simulink model "v2021_10_27_modello_calcolo_trim_1_semplificato"  (R2020b)
settings: Solver=ode4  StartTime=0.0  StopTime=0.01  FixedStep=0.01  RelTol=1e-3
values from neighbouring files (symbols this model uses):
  alphavec_rad = deg2rad(alphavec)    [v2021_10_27_calcoloAerodinamica.m]
  b = 2.62    [v2021_10_27_calcoloAerodinamica.m]
  betavec_rad = deg2rad(betavec)    [v2021_10_27_calcoloAerodinamica.m]
  c = .32    (= 0.32)    [v2021_10_27_calcoloAerodinamica.m]
  cbar = .32    (= 0.32)    [v2021_10_27_calcoloAerodinamica.m]
  CD0 = 0.024    [v2021_10_27_calcoloAerodinamica.m]
  Clp = -0.5058    [v2021_10_27_calcoloAerodinamica.m]
  CLq = 19.166    [v2021_10_27_calcoloAerodinamica.m]
  Clr = 0.1459    [v2021_10_27_calcoloAerodinamica.m]
  Cmq = -81.796    [v2021_10_27_calcoloAerodinamica.m]
  Cnp = 0.007507    [v2021_10_27_calcoloAerodinamica.m]
  Cnr = -1.2593    [v2021_10_27_calcoloAerodinamica.m]
  CYp = 0.050728    [v2021_10_27_calcoloAerodinamica.m]
  CYr = 0.358925    [v2021_10_27_calcoloAerodinamica.m]
  deltaAtrim = 0    [v2021_10_27_avvioSITL.m]
  deltaEtrim = 0    [v2021_10_27_avvioSITL.m]
  deltaRtrim = 0    [v2021_10_27_avvioSITL.m]
  deltaTtrim = 0.1    [v2021_10_27_avvioSITL.m]
  Dprop = 2*Rprop    (= 0.5334)    [v2021_10_27_calcoloAerodinamica.m]
  Jeng = 0    [v2021_10_27_calcoloAerodinamica.m]
  Jprop = mprop*(Dprop^2)/12    (= 0.00422031414)    [v2021_10_27_calcoloAerodinamica.m]
  matricepolinomi = [0.0816560564319 0.0869820125665 0.0279748858868 -4.51852057237 0.0146653626785 -0.925775006168 8.18052218957e-06 -1.47322908992e-05 7.59644694438e-06 0.00246695371279 9.02269223066e-06 0.000559334242525 ... (126 elements, 6x21)]    [coefficienti_curve_renard.mat]
  q = stato(11)    [measure_F1B.m]
  r = stato(12)    [measure_F1B.m]
  rACtG = rACtP-rGP    [v2021_10_27_calcoloAerodinamica.m]
  rACwG = rACwP-rGP    [v2021_10_27_calcoloAerodinamica.m]
  rAHRSG = rAHRSP-rGP    [v2021_10_27_calcoloAerodinamica.m]
  rho = 1.21330    (= 1.2133)    [v2021_10_27_calcoloAerodinamica.m]
  rLEG = rLEP-rGP    [v2021_10_27_calcoloAerodinamica.m]
  rmglG = rmglP-rGP    [v2021_10_27_calcoloAerodinamica.m]
  rmgrG = rmgrP-rGP    [v2021_10_27_calcoloAerodinamica.m]
  rngG = rngP-rGP    [v2021_10_27_calcoloAerodinamica.m]
  rNPG = rNPP-rGP    [v2021_10_27_calcoloAerodinamica.m]
  rPG = -rGP    [v2021_10_27_calcoloAerodinamica.m]
  Rprop = 0.2667    [v2021_10_27_calcoloAerodinamica.m]
  S = b*cbar    (= 0.8384)    [v2021_10_27_calcoloAerodinamica.m]
  W = m*g    [v2021_10_27_calcoloAerodinamica.m]
  Zeng = rPG(3)    [v2021_10_27_calcoloAerodinamica.m]
undefined symbols (not defined in the file or in its folder): CldA, CLdE, CldR, CmdE, CndA, CndR, CYdA, CYdR, F, J_vec, MIL
libraries: aerolibwind2 x3, shared6dof x1, aerolibasang x1, simulink x1
(part 2 of 2)

== system v2021_10_27_modello_calcolo_trim_1_semplificato/AENEA II /Forze aerodinamiche1/Forze assi vento//q/Subsystem2 ==
  note: CL=CL(ALPHA_X,BETA)+CL_q*q+CL_de*de
  q : Inport
  deltaE : Inport  Port=2
  Vect_Costanti : Inport  Port=3
  "Vbpolare " : Inport  Port=4
  2-D Lookup Table : Lookup_n-D  BreakpointsForDimension1=alphavec_rad  BreakpointsForDimension2=betavec_rad  Table=CL(2:end,2:end)  InternalRulePriority=Speed  RndMeth=Simplest  InputSameDT=on
      settings: InputPortMap=u0,u1
  Bus Selector : BusSelector  OutputSignals=Coef_Aerodinamici.Coef_Forze.CLq,Coef_Aerodinamici.Coef_Forze.CLdE,Coef_Geometrici.cbar
  Bus Selector1 : BusSelector  OutputSignals=α,β,V
  Gain1 : Gain  Gain=2
  Mux : Mux
  Product4 : Product
  Sum : Sum  Inputs=3
  "controllo divisione per zero Lq " : MATLAB Function  TreatAsAtomicUnit=on
  CL : Outport  VectorParamsAs1DForOutWhenUnconnected=off
  wires:
  Sum/1 -> CL/1
  q/1 -> Mux/2
  Bus Selector/1 -> Mux/1  "<CLq>"
  Bus Selector/2 -> Product4/1  "<CLdE>"
  deltaE/1 -> Product4/2
  "controllo divisione per zero Lq "/1(y) -> Sum/2
  Product4/1 -> Sum/3
  2-D Lookup Table/1 -> Sum/1
  Vect_Costanti/1 -> Bus Selector/1
  Gain1/1 -> Mux/4
  Bus Selector/3 -> Mux/3  "<cbar>"
  Bus Selector1/1 -> 2-D Lookup Table/1  "<α>"
  "Vbpolare "/1 -> Bus Selector1/1
  Bus Selector1/3 -> Gain1/1  "<V>"
  Bus Selector1/2 -> 2-D Lookup Table/2  "<β>"
  Mux/1 -> "controllo divisione per zero Lq "/1(u)

== system v2021_10_27_modello_calcolo_trim_1_semplificato/AENEA II /Forze aerodinamiche1/Momenti //press din/Subsystem3 ==
  note: Gain aggiunto da CV e FM per modificare il CLBeta
  note: Cl=Cl(alpha_x,beta)+Cl_p*p+Cl_r*r+Cl_dA*dA+Cl_dR*dR
  Vect_Costanti : Inport
  Vect_Comandi : Inport  Port=2
  "Vbpolare " : Inport  Port=3
  ωb : Inport  Port=4
  2-D Lookup Table : Lookup_n-D  BreakpointsForDimension1=alphavec_rad  BreakpointsForDimension2=betavec_rad  Table=Cl(2:end,2:end)  InternalRulePriority=Speed  RndMeth=Simplest  InputSameDT=on
      settings: InputPortMap=u0,u1
  Bus Selector : BusSelector  OutputSignals=Coef_Aerodinamici.Coef_Momenti.Clp,Coef_Geometrici.b/2,Coef_Aerodinamici.Coef_Momenti.Clr,Coef_Aerodinamici.Coef_Momenti.CldA,Coef_Aerodinamici.Coef_Momenti.CldR
  Bus Selector1 : BusSelector  OutputSignals=deltaA,deltaR
  Bus Selector2 : BusSelector  OutputSignals=α,β,V
  Bus Selector3 : BusSelector  OutputSignals=p,r
  Gain4 : Gain  Gain=1.5
  Mux : Mux
  Mux1 : Mux
  Product2 : Product
  Product3 : Product
  Sum : Sum  Inputs=5
  "controllo divisione per zero lp " : MATLAB Function  TreatAsAtomicUnit=on
  "controllo divisione per zero lr " : MATLAB Function  TreatAsAtomicUnit=on
  Cl : Outport  VectorParamsAs1DForOutWhenUnconnected=off
  wires:
  Sum/1 -> Cl/1
  Bus Selector/3 -> Mux1/1  "<Clr>"
  Bus Selector1/2 -> Product3/2  "<deltaR>"
  Bus Selector1/1 -> Product2/2  "<deltaA>"
  Product3/1 -> Sum/5
  Product2/1 -> Sum/4
  "controllo divisione per zero lp "/1(y) -> Sum/2
  2-D Lookup Table/1 -> Gain4/1
  Gain4/1 -> Sum/1
  Vect_Costanti/1 -> Bus Selector/1
  Bus Selector/1 -> Mux/1  "<Clp>"
  Bus Selector/5 -> Product3/1  "<CldR>"
  Bus Selector/4 -> Product2/1  "<CldA>"
  Bus Selector/2 -> Mux1/2, Mux/3  "<b/2>"
  Vect_Comandi/1 -> Bus Selector1/1
  Bus Selector2/1 -> 2-D Lookup Table/1  "<α>"
  "Vbpolare "/1 -> Bus Selector2/1
  Bus Selector2/3 -> Mux1/4, Mux/4  "<V>"
  Bus Selector2/2 -> 2-D Lookup Table/2  "<β>"
  ωb/1 -> Bus Selector3/1
  Bus Selector3/1 -> Mux/2  "<p>"
  Bus Selector3/2 -> Mux1/3  "<r>"
  Mux/1 -> "controllo divisione per zero lp "/1(u)
  Mux1/1 -> "controllo divisione per zero lr "/1(u)
  "controllo divisione per zero lr "/1(y) -> Sum/3

== system v2021_10_27_modello_calcolo_trim_1_semplificato/AENEA II /Forze aerodinamiche1/Momenti //press din/Subsystem4 ==
  note: Cm=Cm(alpha_x,beta)+Cmq*q+Cm_deltaE*deltaE
  Vect_Costanti : Inport
  Vect_Comandi : Inport  Port=2
  "Vbpolare " : Inport  Port=3
  ωb : Inport  Port=4
  2-D Lookup Table : Lookup_n-D  BreakpointsForDimension1=alphavec_rad  BreakpointsForDimension2=betavec_rad  Table=Cm(2:end,2:end)  InternalRulePriority=Speed  RndMeth=Simplest  InputSameDT=on
      settings: InputPortMap=u0,u1
  Bus Selector : BusSelector  OutputSignals=deltaE
  Bus Selector1 : BusSelector  OutputSignals=Coef_Geometrici.cbar,Coef_Aerodinamici.Coef_Momenti.Cmq,Coef_Aerodinamici.Coef_Momenti.CmdE
  Bus Selector2 : BusSelector  OutputSignals=α,β,V
  Bus Selector3 : BusSelector  OutputSignals=q
  Gain1 : Gain  Gain=2
  Mux : Mux
  Product2 : Product
  Sum : Sum  Inputs=3
  "controllo divisione per zero mq " : MATLAB Function  TreatAsAtomicUnit=on
  Cm : Outport  VectorParamsAs1DForOutWhenUnconnected=off
  wires:
  Bus Selector1/2 -> Mux/1  "<Cmq>"
  Sum/1 -> Cm/1
  Gain1/1 -> Mux/4
  Bus Selector1/3 -> Product2/1  "<CmdE>"
  Bus Selector/1 -> Product2/2  "<deltaE>"
  Product2/1 -> Sum/3
  2-D Lookup Table/1 -> Sum/1
  Vect_Comandi/1 -> Bus Selector/1
  Vect_Costanti/1 -> Bus Selector1/1
  Bus Selector1/1 -> Mux/3  "<cbar>"
  Bus Selector2/3 -> Gain1/1  "<V>"
  "Vbpolare "/1 -> Bus Selector2/1
  Bus Selector2/1 -> 2-D Lookup Table/1  "<α>"
  Bus Selector2/2 -> 2-D Lookup Table/2  "<β>"
  ωb/1 -> Bus Selector3/1
  Bus Selector3/1 -> Mux/2  "<q>"
  Mux/1 -> "controllo divisione per zero mq "/1(u)
  "controllo divisione per zero mq "/1(y) -> Sum/2

== system v2021_10_27_modello_calcolo_trim_1_semplificato/AENEA II /Forze aerodinamiche1/Momenti //press din/Subsystem5 ==
  note: Cn=Cn(alpha_x,beta)+Cn_p*p+Cn_r*r+Cn_deltaA*deltaA+Cn_deltaR*deltaR
  Vect_Costanti : Inport
  Vect_Comandi : Inport  Port=2
  "Vbpolare " : Inport  Port=3
  ωb : Inport  Port=4
  2-D Lookup Table : Lookup_n-D  BreakpointsForDimension1=alphavec_rad  BreakpointsForDimension2=betavec_rad  Table=Cn(2:end,2:end)  InternalRulePriority=Speed  RndMeth=Simplest  InputSameDT=on
      settings: InputPortMap=u0,u1
  Bus Selector : BusSelector  OutputSignals=deltaA,deltaR
  Bus Selector1 : BusSelector  OutputSignals=Coef_Aerodinamici.Coef_Momenti.Cnr,Coef_Geometrici.b/2,Coef_Aerodinamici.Coef_Momenti.Cnp,Coef_Aerodinamici.Coef_Momenti.CndA,Coef_Aerodinamici.Coef_Momenti.CndR
  Bus Selector2 : BusSelector  OutputSignals=α,β,V
  Bus Selector3 : BusSelector  OutputSignals=p,q,r
  Mux : Mux
  Mux1 : Mux
  Product2 : Product
  Product3 : Product
  Sum : Sum  Inputs=5
  Terminator : Terminator
  "controllo divisione per zero np " : MATLAB Function  TreatAsAtomicUnit=on
  "controllo divisione per zero nr " : MATLAB Function  TreatAsAtomicUnit=on
  Cn : Outport  VectorParamsAs1DForOutWhenUnconnected=off
  wires:
  Bus Selector1/3 -> Mux1/1  "<Cnp>"
  Product2/1 -> Sum/4
  Product3/1 -> Sum/5
  Sum/1 -> Cn/1
  Bus Selector1/1 -> Mux/1  "<Cnr>"
  Bus Selector1/5 -> Product3/1  "<CndR>"
  Bus Selector/2 -> Product3/2  "<deltaR>"
  Bus Selector/1 -> Product2/2  "<deltaA>"
  2-D Lookup Table/1 -> Sum/1
  Vect_Comandi/1 -> Bus Selector/1
  Vect_Costanti/1 -> Bus Selector1/1
  Bus Selector1/4 -> Product2/1  "<CndA>"
  Bus Selector1/2 -> Mux1/3, Mux/3  "<b/2>"
  Bus Selector2/3 -> Mux1/4, Mux/4  "<V>"
  "Vbpolare "/1 -> Bus Selector2/1
  Bus Selector2/1 -> 2-D Lookup Table/1  "<α>"
  Bus Selector2/2 -> 2-D Lookup Table/2  "<β>"
  ωb/1 -> Bus Selector3/1
  Bus Selector3/3 -> Mux/2  "<r>"
  Bus Selector3/1 -> Mux1/2  "<p>"
  Bus Selector3/2 -> Terminator/1  "<q>"
  Mux/1 -> "controllo divisione per zero nr "/1(u)
  "controllo divisione per zero nr "/1(y) -> Sum/3
  Mux1/1 -> "controllo divisione per zero np "/1(u)
  "controllo divisione per zero np "/1(y) -> Sum/2

== matlab function v2021_10_27_modello_calcolo_trim_1_semplificato/AENEA II /Velocità1/controllo divisione per 0 su alpha ==
  data: u input; y output
function y = tgalpha(u)

if length(u)~=2
    error('vettore ingresso errato')
else
    if u(2)==0
        y=0;
    else 
        y=u(1)/u(2);
    end
end

== matlab function v2021_10_27_modello_calcolo_trim_1_semplificato/AENEA II /Velocità1/controllo divisione per 0 su beta ==
  data: u input; y output
function y = sinbeta(u)

if length(u)~=2
    error('vettore ingresso errato')
else
    if u(2)==0
        y=0;
    else 
        y=u(1)/u(2);
    end
end

== matlab function v2021_10_27_modello_calcolo_trim_1_semplificato/AENEA II /Forze aerodinamiche1/Forze assi vento//q/Subsystem1/controllo divisione per zero Yp  ==
  data: u input; y output
function y = Yp(u)

if length(u)~=4
    error('vettore ingresso dimensione errata')
else
    if u(4)==0
        y=0;
    else
        y=u(1)*u(2)*u(3)/u(4);
    end
end

== matlab function v2021_10_27_modello_calcolo_trim_1_semplificato/AENEA II /Forze aerodinamiche1/Forze assi vento//q/Subsystem1/controllo divisione per zero Yr ==
  data: u input; y output
function y = Yr(u)

if length(u)~=4
    error('vettore ingresso dimensione errata')
else
    if u(4)==0
        y=0;
    else
        y=u(1)*u(2)*u(3)/u(4);
    end
end

== matlab function v2021_10_27_modello_calcolo_trim_1_semplificato/AENEA II /Forze aerodinamiche1/Forze assi vento//q/Subsystem2/controllo divisione per zero Lq  ==
  data: u input; y output
function y = Lq(u)

if length(u)~=4
    error('vettore ingresso dimensione errata')
else
    if u(4)==0
        y=0;
    else
        y=u(1)*u(2)*u(3)/u(4);
    end
end

== matlab function v2021_10_27_modello_calcolo_trim_1_semplificato/AENEA II /Forze aerodinamiche1/MATLAB Function ==
  data: alpha input; Lbw output; beta input
function Lbw = DCMbw(alpha,beta)


Lbw=[cos(alpha)*cos(beta), -cos(alpha)*sin(beta), -sin(alpha); sin(beta), cos(beta), 0; sin(alpha)*cos(beta), -sin(alpha)*sin(beta), cos(alpha)];

== matlab function v2021_10_27_modello_calcolo_trim_1_semplificato/AENEA II /Forze aerodinamiche1/Momenti //press din/Subsystem3/controllo divisione per zero lp  ==
  data: u input; y output
function y = lp(u)

if length(u)~=4
    error('vettore ingresso dimensione errata')
else
    if u(4)==0
        y=0;
    else
        y=u(1)*u(2)*u(3)/u(4);
    end
end

== matlab function v2021_10_27_modello_calcolo_trim_1_semplificato/AENEA II /Forze aerodinamiche1/Momenti //press din/Subsystem3/controllo divisione per zero lr  ==
  data: u input; y output
function y = lr(u)

if length(u)~=4
    error('vettore ingresso dimensione errata')
else
    if u(4)==0
        y=0;
    else
        y=u(1)*u(2)*u(3)/u(4);
    end
end

== matlab function v2021_10_27_modello_calcolo_trim_1_semplificato/AENEA II /Forze aerodinamiche1/Momenti //press din/Subsystem4/controllo divisione per zero mq  ==
  data: u input; y output
function y = mq(u)

if length(u)~=4
    error('vettore ingresso dimensione errata')
else
    if u(4)==0
        y=0;
    else
        y=u(1)*u(2)*u(3)/u(4);
    end
end

== matlab function v2021_10_27_modello_calcolo_trim_1_semplificato/AENEA II /Forze aerodinamiche1/Momenti //press din/Subsystem5/controllo divisione per zero np  ==
  data: u input; y output
function y = np(u)

if length(u)~=4
    error('vettore ingresso dimensione errata')
else
    if u(4)==0
        y=0;
    else
        y=u(1)*u(2)*u(3)/u(4);
    end
end

== matlab function v2021_10_27_modello_calcolo_trim_1_semplificato/AENEA II /MATLAB Function ==
  data: PHI input; invR output
function invR = omega2PHIdot(PHI)

if length(PHI)==3
    Phi=PHI(1);
    Theta=PHI(2);
    
    invR=[1, sin(Phi)*tan(Theta), cos(Phi)*tan(Theta); 0, cos(Phi), -sin(Phi); 0, sin(Phi)*sec(Theta), cos(Phi)*sec(Theta)];
else 
    error('il vettore PHI non va bene')
end

== matlab function v2021_10_27_modello_calcolo_trim_1_semplificato/AENEA II /Forze aerodinamiche1/Momenti //press din/Subsystem5/controllo divisione per zero nr  ==
  data: u input; y output
function y = nr(u)

if length(u)~=4
    error('vettore ingresso dimensione errata')
else
    if u(4)==0
        y=0;
    else
        y=u(1)*u(2)*u(3)/u(4);
    end
end

== matlab function v2021_10_27_modello_calcolo_trim_1_semplificato/AENEA II /Propulsione1/LUT ELICA 1/MATLAB Function ==
  data: J input; Ct output; RPM input; Cp output; matricepolinomi input
function [Ct,Cp] = calcolo_Ct_Cp(J,RPM,matricepolinomi)

lct00 = matricepolinomi(1,1);
lct10 = matricepolinomi(1,2);
lct01 = matricepolinomi(1,3);
lct20 = matricepolinomi(1,4);
lct11 = matricepolinomi(1,5);
lct02 = matricepolinomi(1,6);
lct30 = matricepolinomi(1,7);
lct21 = matricepolinomi(1,8);
lct12 = matricepolinomi(1,9);
lct40 = matricepolinomi(1,10);
lct31 = matricepolinomi(1,11);
lct22 = matricepolinomi(1,12);

qct00 = matricepolinomi(2,1);
qct10 = matricepolinomi(2,2);
qct01 = matricepolinomi(2,3);
qct20 = matricepolinomi(2,4);
qct11 = matricepolinomi(2,5);
qct02 = matricepolinomi(2,6);
qct30 = matricepolinomi(2,7);
qct21 = matricepolinomi(2,8);
qct12 = matricepolinomi(2,9);
qct03 = matricepolinomi(2,10);
qct40 = matricepolinomi(2,11);
qct31 = matricepolinomi(2,12);
qct22 = matricepolinomi(2,13);
qct13 = matricepolinomi(2,14);
qct04 = matricepolinomi(2,15);
qct50 = matricepolinomi(2,16);
qct41 = matricepolinomi(2,17);
qct32 = matricepolinomi(2,18);
qct23 = matricepolinomi(2,19);
qct14 = matricepolinomi(2,20);
qct05 = matricepolinomi(2,21);

cp100 = matricepolinomi(3,1);
cp110 = matricepolinomi(3,2);
cp101 = matricepolinomi(3,3);
cp120 = matricepolinomi(3,4);
cp111 = matricepolinomi(3,5);
cp102 = matricepolinomi(3,6);
cp130 = matricepolinomi(3,7);
cp121 = matricepolinomi(3,8);
cp112 = matricepolinomi(3,9);
cp140 = matricepolinomi(3,10);
cp131 = matricepolinomi(3,11);
cp122 = matricepolinomi(3,12);

cp200 = matricepolinomi(4,1);
cp210 = matricepolinomi(4,2);
cp201 = matricepolinomi(4,3);
cp220 = matricepolinomi(4,4);
cp211 = matricepolinomi(4,5);
cp202 = matricepolinomi(4,6);
cp230 = matricepolinomi(4,7);
cp221 = matricepolinomi(4,8);
cp212 = matricepolinomi(4,9);
cp240 = matricepolinomi(4,10);
cp231 = matricepolinomi(4,11);
cp222 = matricepolinomi(4,12);

cp300 = matricepolinomi(5,1);
cp310 = matricepolinomi(5,2);
cp301 = matricepolinomi(5,3);
cp320 = matricepolinomi(5,4);
cp311 = matricepolinomi(5,5);
cp302 = matricepolinomi(5,6);
cp330 = matricepolinomi(5,7);
cp321 = matricepolinomi(5,8);
cp312 = matricepolinomi(5,9);
cp340 = matricepolinomi(5,10);
cp331 = matricepolinomi(5,11);
cp322 = matricepolinomi(5,12);

cp400 = matricepolinomi(6,1);
cp410 = matricepolinomi(6,2);
cp401 = matricepolinomi(6,3);
cp420 = matricepolinomi(6,4);
cp411 = matricepolinomi(6,5);
cp402 = matricepolinomi(6,6);
cp430 = matricepolinomi(6,7);
cp421 = matricepolinomi(6,8);
cp412 = matricepolinomi(6,9);
cp440 = matricepolinomi(6,10);
cp431 = matricepolinomi(6,11);
cp422 = matricepolinomi(6,12);


if J<=0.32
    x = RPM;
    y = J;
    Ct = qct00 + qct10*x + qct01*y + qct20*x^2 + qct11*x*y + qct02*y^2 + qct30*x^3 + qct21*x^2*y + qct12*x*y^2 + qct03*y^3 + qct40*x^4 + qct31*x^3*y + qct22*x^2*y^2 + qct13*x*y^3 + qct04*y^4 + qct50*x^5 + qct41*x^4*y + qct32*x^3*y^2 + qct23*x^2*y^3 + qct14*x*y^4 + qct05*y^5;
elseif J>0.32
    x = RPM;
    y = J;
    Ct = lct00 + lct10*x + lct01*y + lct20*x^2 + lct11*x*y + lct02*y^2 + lct30*x^3 + lct21*x^2*y + lct12*x*y^2 + lct40*x^4 + lct31*x^3*y + lct22*x^2*y^2;
else
    Ct = 0;
end

if (J<=0.34)&&(RPM<=5000)
    x = RPM;
    y = J;
    Cp = cp100 + cp110*x + cp101*y + cp120*x^2 + cp111*x*y + cp102*y^2 + cp130*x^3 + cp121*x^2*y + cp112*x*y^2 + cp140*x^4 + cp131*x^3*y + cp122*x^2*y^2;
elseif (J<=0.34)&&(RPM>5000)
    x = RPM;
    y = J;
    Cp = cp200 + cp210*x + cp201*y + cp220*x^2 + cp211*x*y + cp202*y^2 + cp230*x^3 + cp221*x^2*y + cp212*x*y^2 + cp240*x^4 + cp231*x^3*y + cp222*x^2*y^2;
elseif (J>0.34)&&(RPM<=5000)
    x = RPM;
    y = J;
    Cp = cp300 + cp310*x + cp301*y + cp320*x^2 + cp311*x*y + cp302*y^2 + cp330*x^3 + cp321*x^2*y + cp312*x*y^2 + cp340*x^4 + cp331*x^3*y + cp322*x^2*y^2;
elseif (J>0.34)&&(RPM>5000)
    x = RPM;
    y = J;
    Cp = cp400 + cp410*x + cp401*y + cp420*x^2 + cp411*x*y + cp402*y^2 + cp430*x^3 + cp421*x^2*y + cp412*x*y^2 + cp440*x^4 + cp431*x^3*y + cp422*x^2*y^2;
else
    Cp = 0;
end

== matlab function v2021_10_27_modello_calcolo_trim_1_semplificato/AENEA II /Velocità2/MATLAB Function ==
  data: V input; module output
function module = absolute(V)

module=sqrt((V(1)^2)+(V(2)^2)+(V(3)^2));

end

== matlab function v2021_10_27_modello_calcolo_trim_1_semplificato/AENEA II /Velocità2/controllo divisione per 0 su alpha ==
  data: u input; y output
function y = tgalpha(u)

if length(u)~=2
    error('vettore ingresso errato')
else
    if u(2)==0
        y=0;
    else 
        y=u(1)/u(2);
    end
end

== matlab function v2021_10_27_modello_calcolo_trim_1_semplificato/AENEA II /Velocità2/controllo divisione per 0 su beta ==
  data: u input; y output
function y = sinbeta(u)

if length(u)~=2
    error('vettore ingresso errato')
else
    if u(2)==0
        y=0;
    else 
        y=u(1)/u(2);
    end
end

== matlab function v2021_10_27_modello_calcolo_trim_1_semplificato/AENEA II /Velocità2/MATLAB Function1 ==
  data: V input; module output
function module = absolute(V)

module=sqrt((V(1)^2)+(V(2)^2)+(V(3)^2));

end

== matlab function v2021_10_27_modello_calcolo_trim_1_semplificato/AENEA II /Forze aerodinamiche/MATLAB Function ==
  data: alpha input; Lbw output; beta input
function Lbw = DCMbw(alpha,beta)


Lbw=[cos(alpha)*cos(beta), -cos(alpha)*sin(beta), -sin(alpha); sin(beta), cos(beta), 0; sin(alpha)*cos(beta), -sin(alpha)*sin(beta), cos(alpha)];

== matlab function v2021_10_27_modello_calcolo_trim_1_semplificato/AENEA II /Forze aerodinamiche/Forze assi vento//q/Subsystem1/controllo divisione per zero Yp  ==
  data: u input; y output
function y = Yp(u)

if length(u)~=4
    error('vettore ingresso dimensione errata')
else
    if u(4)==0
        y=0;
    else
        y=u(1)*u(2)*u(3)/u(4);
    end
end

== matlab function v2021_10_27_modello_calcolo_trim_1_semplificato/AENEA II /Forze aerodinamiche/Forze assi vento//q/Subsystem1/controllo divisione per zero Yr ==
  data: u input; y output
function y = Yr(u)

if length(u)~=4
    error('vettore ingresso dimensione errata')
else
    if u(4)==0
        y=0;
    else
        y=u(1)*u(2)*u(3)/u(4);
    end
end

== matlab function v2021_10_27_modello_calcolo_trim_1_semplificato/AENEA II /Forze aerodinamiche/Forze assi vento//q/Subsystem2/controllo divisione per zero Lq  ==
  data: u input; y output
function y = Lq(u)

if length(u)~=4
    error('vettore ingresso dimensione errata')
else
    if u(4)==0
        y=0;
    else
        y=u(1)*u(2)*u(3)/u(4);
    end
end

== matlab function v2021_10_27_modello_calcolo_trim_1_semplificato/AENEA II /Forze aerodinamiche/Momenti //press din/Subsystem3/controllo divisione per zero lp  ==
  data: u input; y output
function y = lp(u)

if length(u)~=4
    error('vettore ingresso dimensione errata')
else
    if u(4)==0
        y=0;
    else
        y=u(1)*u(2)*u(3)/u(4);
    end
end

== matlab function v2021_10_27_modello_calcolo_trim_1_semplificato/AENEA II /Forze aerodinamiche/Momenti //press din/Subsystem3/controllo divisione per zero lr  ==
  data: u input; y output
function y = lr(u)

if length(u)~=4
    error('vettore ingresso dimensione errata')
else
    if u(4)==0
        y=0;
    else
        y=u(1)*u(2)*u(3)/u(4);
    end
end

== matlab function v2021_10_27_modello_calcolo_trim_1_semplificato/AENEA II /Forze aerodinamiche/Momenti //press din/Subsystem4/controllo divisione per zero mq  ==
  data: u input; y output
function y = mq(u)

if length(u)~=4
    error('vettore ingresso dimensione errata')
else
    if u(4)==0
        y=0;
    else
        y=u(1)*u(2)*u(3)/u(4);
    end
end

== matlab function v2021_10_27_modello_calcolo_trim_1_semplificato/AENEA II /Forze aerodinamiche/Momenti //press din/Subsystem5/controllo divisione per zero nr  ==
  data: u input; y output
function y = nr(u)

if length(u)~=4
    error('vettore ingresso dimensione errata')
else
    if u(4)==0
        y=0;
    else
        y=u(1)*u(2)*u(3)/u(4);
    end
end

== matlab function v2021_10_27_modello_calcolo_trim_1_semplificato/AENEA II /Forze aerodinamiche/Momenti //press din/Subsystem5/controllo divisione per zero np  ==
  data: u input; y output
function y = np(u)

if length(u)~=4
    error('vettore ingresso dimensione errata')
else
    if u(4)==0
        y=0;
    else
        y=u(1)*u(2)*u(3)/u(4);
    end
end

== matlab function v2021_10_27_modello_calcolo_trim_1_semplificato/AENEA II /Velocità1/MATLAB Function ==
  data: V input; module output
function module = absolute(V)


if length(V)==3
   module=sqrt((V(1)^2)+(V(2)^2)+(V(3)^2));
else 
    error('dimension of input incorrect')
end
